simulink model "ROPOD_4Wheel_Tdistkinb_cntr"  (R2017b)
settings: Solver=ode1  StartTime=0.0  StopTime=Tfinal  FixedStep=Ts  RelTol=1e-3  EnableMultiTasking=on
PreLoadFcn:
  | init_model
InitFcn:
  | init_model
values from neighbouring files (symbols this model uses):
  FFtheta_intia = 0    [init_model.m]
  FFxy_mass = 0*80    (= 0)    [init_model.m]
  I_fhz_dtheta_cntr = 0.3    [init_model.m]
  I_fhz_dxdy_cntr = 0.25    [init_model.m]
  K_gain_dtheta_cntr = 150    [init_model.m]
  K_gain_dxdy_cntr = 200    [init_model.m]
  LL_wp_fhz_dtheta_cntr = 20    [init_model.m]
  LL_wp_fhz_dxdy_cntr = 20    [init_model.m]
  LL_wz_fhz_dtheta_cntr = 20    [init_model.m]
  LL_wz_fhz_dxdy_cntr = 20    [init_model.m]
  LPF_fhz_ddelta_meas = 50    [init_model.m]
  LPF_fhz_dtheta_cntr = 100    [init_model.m]
  LPF_fhz_dvarphi_meas = 50    [init_model.m]
  LPF_fhz_dxdy_cntr = 100    [init_model.m]
  max_hw_tau = 7.0    (= 7)    [init_model.m]
  max_ropod_acc_theta = 1.6    [init_model.m]
  max_ropod_acc_xy = 2.0    (= 2)    [init_model.m]
  max_ropod_sw_force = 500    [init_model.m]
  max_ropod_sw_tau = 250    [init_model.m]
  max_ropod_vel_theta = 1.6    [init_model.m]
  max_ropod_vel_xy = 2.0    (= 2)    [init_model.m]
  max_sw_current = 10    [init_model.m]
  Nwheels = 4    [Jqwl_numeric_function.m]    (also in S_matrix.m; extract_kinmodel_parameters.m; init_model.m; tau_optimal_dist_vec_fun.m)
  pivot_offs_sws = [3.835 3.465 2.059 0.357]    [init_model.m]
  ropod_kinmodel_pv = struct2array(ropod_kinmodel_param)    [set_ropod_KinModparams.m]
  SW_COM1_ENABLE1 = hex2dec('0001')    [init_model.m]
  SW_COM1_ENABLE2 = hex2dec('0002')    [init_model.m]
  SW_COM1_MODE_TORQUE = bitshift(hex2dec('0000'),2)    [init_model.m]
  SW_COM1_MODE_VELOCITY = bitshift(hex2dec('0002'),2)    [init_model.m]
  SW_COM1_USE_TS = hex2dec('8000')    [init_model.m]
  sw_tau_2_curr = 1/motor_physical_parameters.torqueconstant.value    [init_model.m]
  Taucompfactor = 2.0    (= 2)    [init_model.m]
  Tinit = 0*Tslot    [init_model.m]
  Ts = 0.001    [init_model.m]
undefined symbols (not defined in the file or in its folder): DiscIntNeverNeededParam, I_fhz_dvarphi_cntr, K_gain_dvarphi_cntr, LL_wp_fhz_dvarphi_cntr, LL_wz_fhz_dvarphi_cntr, LPF_fhz_dvarphi_cntr
libraries: simulink x37, cstblocks x23, dspsigops x12, SOEM_EtherCAT_Lib x5
(part 1 of 3)
settings Model: SimulationMode=external  Creator=cesar  LastModifiedBy=cesar
settings OptimizationCC: PassReuseOutputArgsThreshold=0  MaxStackSize=64
settings DebuggingCC: ParameterTunabilityLossMsg=error
settings HardwareCC: ProdBitPerLong=64  ProdHWDeviceType=Intel->x86-64 (Linux 64)  TargetBitPerLong=64  TargetBitPerPointer=64  TargetBitPerSizeT=64  TargetBitPerPtrDiffT=64  TargetLargestAtomicFloat=Float  TargetIntDivRoundTo=Zero  TargetEndianess=LittleEndian  TargetWordSize=64  TargetHWDeviceType=Intel->x86-64 (Linux 64)
settings SFSimCC: MATLABDynamicMemAlloc=off
settings RTWCC: SystemTargetFile=mttarget.tlc  MakeCommand="make_rtw  CC=\"ccache gcc\" OPTS=\"-DNETIF_ID=0 -DTEST_CONN_MODEL -D_GNU_SOURCE -DPRIO=99\""  TemplateMakefile=mt_unix.tmf  Description=Generic Real-Time Target  CustomInclude=/usr/local/include/soem  CustomLibrary=/usr/local/lib/libsoem.so  Toolchain=Catkin  BuildConfiguration=Faster Runs  RTWCompilerOptimization=Custom  RTWCustomCompilerOptimizations=-O2 -g -W
settings CodeAppCC: ForceParamTrailComments=on  OperatorAnnotations=on
settings GRTTargetCC: TargetLangStandard=C89/C90 (ANSI)  UseToolchainInfoCompliant=off  ExtMode=on

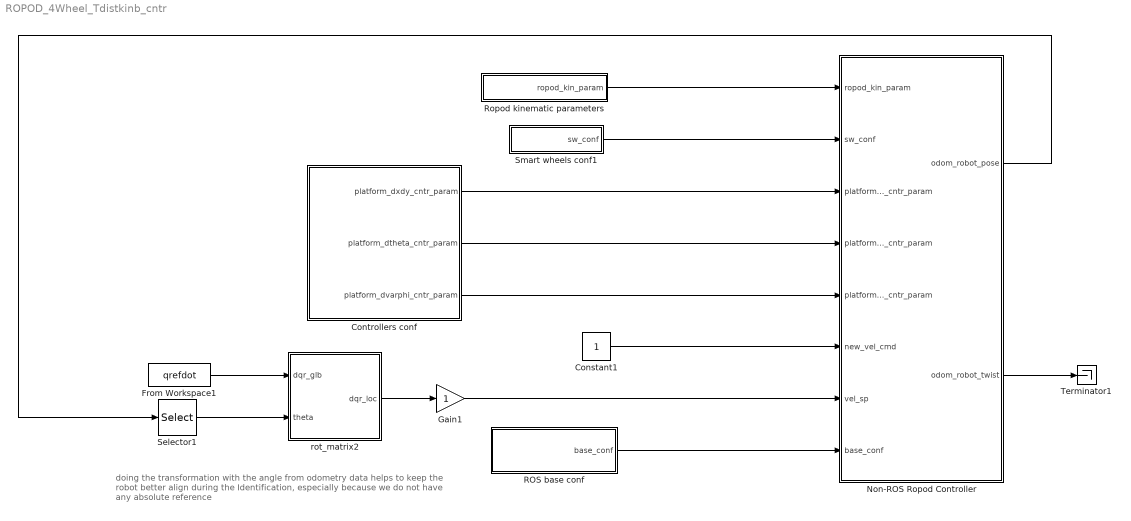
== system ROPOD_4Wheel_Tdistkinb_cntr ==
  note: doing the transformation with the angle from odometry data helps
      | to keep the robot better align during the Identification, especially because
      | we do not have any absolute reference
  Constant1 : Constant
  Controllers conf : Subsystem
  From Workspace1 : FromWorkspace  VariableName=qrefdot  SampleTime=0
  Gain1 : Gain
  Non-ROS Ropod Controller : Subsystem
  ROS base conf : Subsystem
  Ropod kinematic parameters : Subsystem
  Selector1 : Selector  InputPortWidth=3  IndexOptions=Index vector (dialog)  Indices=3  OutputSizes=1
  Smart wheels conf1 : Subsystem
  Terminator1 : Terminator
  rot_matrix2 : MATLAB Function  TreatAsAtomicUnit=on
  wires:
  Non-ROS Ropod Controller/1(odom_robot_pose) -> Selector1/1
  Gain1/1 -> Non-ROS Ropod Controller/7(vel_sp)
  ROS base conf/1(base_conf) -> Non-ROS Ropod Controller/8(base_conf)
  Non-ROS Ropod Controller/2(odom_robot_twist) -> Terminator1/1
  Constant1/1 -> Non-ROS Ropod Controller/6(new_vel_cmd)
  Controllers conf/1(platform_dxdy_cntr_param) -> Non-ROS Ropod Controller/3(platform_dxdy_cntr_param)
  Smart wheels conf1/1(sw_conf) -> Non-ROS Ropod Controller/2(sw_conf)
  Ropod kinematic parameters/1(ropod_kin_param) -> Non-ROS Ropod Controller/1(ropod_kin_param)
  From Workspace1/1 -> rot_matrix2/1(dqr_glb)
  Controllers conf/3(platform_dvarphi_cntr_param) -> Non-ROS Ropod Controller/5(platform_dvarphi_cntr_param)
  rot_matrix2/1(dqr_loc) -> Gain1/1
  Selector1/1 -> rot_matrix2/2(theta)
  Controllers conf/2(platform_dtheta_cntr_param) -> Non-ROS Ropod Controller/4(platform_dtheta_cntr_param)

== system ROPOD_4Wheel_Tdistkinb_cntr/Controllers conf ==
  Bus Creator : BusCreator  Inputs=5
  Bus Creator1 : BusCreator  Inputs=5
  Bus Creator2 : BusCreator  Inputs=5
  Constant1 : Constant  Value=I_fhz_dxdy_cntr
  Constant10 : Constant  Value=K_gain_dtheta_cntr
  Constant11 : Constant  Value=K_gain_dvarphi_cntr
  Constant12 : Constant  Value=I_fhz_dvarphi_cntr
  Constant13 : Constant  Value=LL_wp_fhz_dvarphi_cntr
  Constant14 : Constant  Value=LL_wz_fhz_dvarphi_cntr
  Constant15 : Constant  Value=LPF_fhz_dvarphi_cntr
  Constant2 : Constant  Value=LL_wp_fhz_dxdy_cntr
  Constant3 : Constant  Value=LL_wz_fhz_dxdy_cntr
  Constant4 : Constant  Value=LPF_fhz_dxdy_cntr
  Constant5 : Constant  Value=I_fhz_dtheta_cntr
  Constant6 : Constant  Value=LL_wp_fhz_dtheta_cntr
  Constant7 : Constant  Value=K_gain_dxdy_cntr
  Constant8 : Constant  Value=LL_wz_fhz_dtheta_cntr
  Constant9 : Constant  Value=LPF_fhz_dtheta_cntr
  platform_dxdy_cntr_param : Outport
  platform_dtheta_cntr_param : Outport  Port=2
  platform_dvarphi_cntr_param : Outport  Port=3
  wires:
  Constant2/1 -> Bus Creator/4  "LL_pole_fhz"
  Constant4/1 -> Bus Creator/5  "LPF_fhz"
  Bus Creator/1 -> platform_dxdy_cntr_param/1
  Constant1/1 -> Bus Creator/2  "I_freq_hz"
  Constant3/1 -> Bus Creator/3  "LL_zero_fhz"
  Constant7/1 -> Bus Creator/1  "P_gain"
  Bus Creator1/1 -> platform_dtheta_cntr_param/1
  Bus Creator2/1 -> platform_dvarphi_cntr_param/1
  Constant5/1 -> Bus Creator1/2  "I_freq_hz"
  Constant6/1 -> Bus Creator1/4  "LL_pole_fhz"
  Constant10/1 -> Bus Creator1/1  "P_gain"
  Constant8/1 -> Bus Creator1/3  "LL_zero_fhz"
  Constant9/1 -> Bus Creator1/5  "LPF_fhz"
  Constant15/1 -> Bus Creator2/5  "LPF_fhz"
  Constant12/1 -> Bus Creator2/2  "I_freq_hz"
  Constant14/1 -> Bus Creator2/3  "LL_zero_fhz"
  Constant11/1 -> Bus Creator2/1  "P_gain"
  Constant13/1 -> Bus Creator2/4  "LL_pole_fhz"

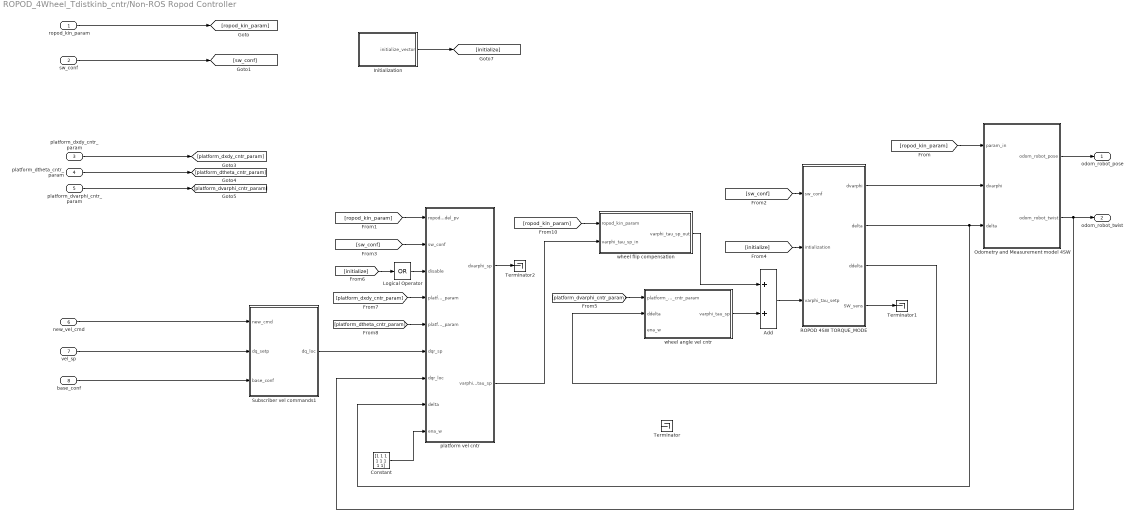
== system ROPOD_4Wheel_Tdistkinb_cntr/Non-ROS Ropod Controller ==
  ropod_kin_param : Inport
  sw_conf : Inport  Port=2
  platform_dxdy_cntr_param : Inport  Port=3
  platform_dtheta_cntr_param : Inport  Port=4
  platform_dvarphi_cntr_param : Inport  Port=5
  new_vel_cmd : Inport  Port=6
  vel_sp : Inport  Port=7
  base_conf : Inport  Port=8
  Add : Sum
  Constant : Constant  Value=[1 1 1 1 1 1 1 1]
  Initialization : Subsystem
  Logical Operator : Logic  Operator=OR  Inputs=1  AllPortsSameDT=off  OutDataTypeStr=boolean
  Odometry and Measurement model 4SW : Subsystem
  ROPOD 4SW TORQUE_MODE : Subsystem
  Subscriber vel commands1 : Subsystem
  Terminator : Terminator
  Terminator1 : Terminator
  Terminator2 : Terminator
  platform vel cntr : Subsystem
  wheel angle vel cntr : Subsystem
  wheel flip compensation : Subsystem
  odom_robot_pose : Outport
  odom_robot_twist : Outport  Port=2
  wires:
  sw_conf/1 -> [sw_conf]
  platform_dvarphi_cntr_param/1 -> [platform_dvarphi_cntr_param]
  platform_dxdy_cntr_param/1 -> [platform_dxdy_cntr_param]
  ropod_kin_param/1 -> [ropod_kin_param]
  platform_dtheta_cntr_param/1 -> [platform_dtheta_cntr_param]
  [ropod_kin_param] -> platform vel cntr/1(ropod_kinmodel_pv)
  Add/1 -> ROPOD 4SW TORQUE_MODE/3(varphi_tau_setp)
  ROPOD 4SW TORQUE_MODE/2(delta) -> platform vel cntr/8(delta), Odometry and Measurement model 4SW/3(delta)
  vel_sp/1 -> Subscriber vel commands1/2(dq_setp)
  ROPOD 4SW TORQUE_MODE/3(ddelta) -> wheel angle vel cntr/2(ddelta)
  [initialize] -> Logical Operator/1
  platform vel cntr/2(varphi_tau_sp) -> wheel flip compensation/2(varphi_tau_sp_in)
  Odometry and Measurement model 4SW/2(odom_robot_twist) -> odom_robot_twist/1, platform vel cntr/7(dqr_loc)
  [sw_conf] -> ROPOD 4SW TORQUE_MODE/1(sw_conf)
  Subscriber vel commands1/1(dq_loc) -> platform vel cntr/6(dqr_sp)
  ROPOD 4SW TORQUE_MODE/4(SW_sens) -> Terminator1/1
  base_conf/1 -> Subscriber vel commands1/3(base_conf)
  ROPOD 4SW TORQUE_MODE/1(dvarphi) -> Odometry and Measurement model 4SW/2(dvarphi)
  [ropod_kin_param] -> Odometry and Measurement model 4SW/1(param_in)
  Constant/1 -> platform vel cntr/9(ena_w)
  Odometry and Measurement model 4SW/1(odom_robot_pose) -> odom_robot_pose/1
  new_vel_cmd/1 -> Subscriber vel commands1/1(new_cmd)
  [platform_dtheta_cntr_param] -> platform vel cntr/5(platform_dtheta_cntr_param)
  [platform_dxdy_cntr_param] -> platform vel cntr/4(platform_dxdy_cntr_param)
  [sw_conf] -> platform vel cntr/2(sw_conf)
  [initialize] -> ROPOD 4SW TORQUE_MODE/2(intialization)
  Initialization/1(initialize_vector) -> [initialize]
  Logical Operator/1 -> platform vel cntr/3(disable)
  platform vel cntr/1(dvarphi_sp) -> Terminator2/1
  wheel angle vel cntr/1(varphi_tau_sp) -> Add/2
  [ropod_kin_param] -> wheel flip compensation/1(ropod_kin_param)
  wheel flip compensation/1(varphi_tau_sp_out) -> Add/1
  [platform_dvarphi_cntr_param] -> wheel angle vel cntr/1(platform_ddelta_cntr_param)

== system ROPOD_4Wheel_Tdistkinb_cntr/ROS base conf ==
  Bus Creator : BusCreator  Inputs=4
  max_ropod_acc_theta : Constant  Value=max_ropod_acc_theta
  max_ropod_acc_xy : Constant  Value=max_ropod_acc_xy
  max_ropod_vel_theta : Constant  Value=max_ropod_vel_theta
  max_ropod_vel_xy : Constant  Value=max_ropod_vel_xy
  base_conf : Outport
  wires:
  max_ropod_acc_xy/1 -> Bus Creator/2  "max_acc_xy"
  max_ropod_vel_xy/1 -> Bus Creator/1  "max_vel_xy"
  Bus Creator/1 -> base_conf/1
  max_ropod_acc_theta/1 -> Bus Creator/4  "max_acc_theta"
  max_ropod_vel_theta/1 -> Bus Creator/3  "max_vel_theta"

== system ROPOD_4Wheel_Tdistkinb_cntr/Ropod kinematic parameters ==
  ropod_kinmodel_pv : Constant  Value=ropod_kinmodel_pv
  ropod_kin_param : Outport
  wires:
  ropod_kinmodel_pv/1 -> ropod_kin_param/1

== system ROPOD_4Wheel_Tdistkinb_cntr/Smart wheels conf1 ==
  Bus Creator : BusCreator  Inputs=8
  LPF_fhz_ddelta_meas : Constant  Value=LPF_fhz_ddelta_meas
  LPF_fhz_dvarphi_meas : Constant  Value=LPF_fhz_dvarphi_meas
  enable : Constant
  max_current : Constant  Value=max_sw_current
  pivot_offset_sw1 : Constant  Value=pivot_offs_sws(1)
  pivot_offset_sw2 : Constant  Value=pivot_offs_sws(2)
  pivot_offset_sw3 : Constant  Value=pivot_offs_sws(3)
  pivot_offset_sw4 : Constant  Value=pivot_offs_sws(4)
  sw_conf : Outport
  wires:
  enable/1 -> Bus Creator/1  "enable"
  Bus Creator/1 -> sw_conf/1
  max_current/1 -> Bus Creator/2  "max_current"
  pivot_offset_sw1/1 -> Bus Creator/3  "pivot_offs_sw1"
  pivot_offset_sw2/1 -> Bus Creator/4  "pivot_offs_sw2"
  pivot_offset_sw3/1 -> Bus Creator/5  "pivot_offs_sw3"
  pivot_offset_sw4/1 -> Bus Creator/6  "pivot_offs_sw4"
  LPF_fhz_dvarphi_meas/1 -> Bus Creator/7  "dvarphi_LPF_fhz"
  LPF_fhz_ddelta_meas/1 -> Bus Creator/8  "ddelta_LPF_fhz"

== system ROPOD_4Wheel_Tdistkinb_cntr/Non-ROS Ropod Controller/Initialization ==
  note: Allow Tinit/Nwheels seconds for initialization per wheel
  Digital Clock : DigitalClock  SampleTime=Ts
  Logical Operator : Logic  AllPortsSameDT=off  OutDataTypeStr=boolean
  Logical Operator1 : Logic  Operator=NOT  AllPortsSameDT=off  OutDataTypeStr=boolean
  Logical Operator2 : Logic  Operator=NOT  AllPortsSameDT=off  OutDataTypeStr=boolean
  Logical Operator3 : Logic  AllPortsSameDT=off  OutDataTypeStr=boolean
  Logical Operator4 : Logic  Operator=NOT  AllPortsSameDT=off  OutDataTypeStr=boolean
  Logical Operator5 : Logic  AllPortsSameDT=off  OutDataTypeStr=boolean
  Mux : Mux
  comp : simulink/Logic and Bit Operations/Compare To Constant  relop=<  const=Tinit/Nwheels  OutDataTypeStr=boolean
  comp1 : simulink/Logic and Bit Operations/Compare To Constant  relop=<  const=2*Tinit/Nwheels  OutDataTypeStr=boolean
  comp2 : simulink/Logic and Bit Operations/Compare To Constant  relop=<  const=3*Tinit/Nwheels  OutDataTypeStr=boolean
  comp3 : simulink/Logic and Bit Operations/Compare To Constant  relop=<  const=4*Tinit/Nwheels  OutDataTypeStr=boolean
  initialize_vector : Outport
  wires:
  Logical Operator5/1 -> Mux/4
  Logical Operator3/1 -> Mux/3
  comp3/1 -> Logical Operator5/2
  Logical Operator2/1 -> Logical Operator3/1
  Logical Operator1/1 -> Logical Operator/1
  Logical Operator4/1 -> Logical Operator5/1
  Mux/1 -> initialize_vector/1
  comp/1 -> Logical Operator1/1, Mux/1
  comp1/1 -> Logical Operator2/1, Logical Operator/2
  Logical Operator/1 -> Mux/2
  comp2/1 -> Logical Operator4/1, Logical Operator3/2
  Digital Clock/1 -> comp3/1, comp2/1, comp1/1, comp/1

== system ROPOD_4Wheel_Tdistkinb_cntr/Non-ROS Ropod Controller/Odometry and Measurement model 4SW ==
  note: This output is only useful when using ros
      | This data is fed to /odom/pose
  note: This part is in global coordinates
  note: This part is in local coordinates
  param_in : Inport
  dvarphi : Inport  Port=2
  delta : Inport  Port=3
  Discrete-Time Integrator : DiscreteIntegrator  InitialConditionSetting=State (most efficient)  SampleTime=Ts  ICPrevOutput=DiscIntNeverNeededParam  ICPrevScaledInput=DiscIntNeverNeededParam
  Jqwl_matrix : MATLAB Function  TreatAsAtomicUnit=on
  Product3 : Product  Multiplication=Matrix(*)
  Selector3 : Selector  InputPortWidth=3  IndexOptions=Index vector (dialog)  Indices=3  OutputSizes=1
  Signal Specification : SignalSpecification  Dimensions=[3 1]
  pos_rot_matrix : MATLAB Function  TreatAsAtomicUnit=on
  odom_robot_pose : Outport
  odom_robot_twist : Outport  Port=2
  wires:
  Product3/1 -> Signal Specification/1
  param_in/1 -> Jqwl_matrix/1(ropod_kinmodel_param_vec)
  delta/1 -> Jqwl_matrix/2(delta)
  Jqwl_matrix/1(Jqwl) -> Product3/1
  dvarphi/1 -> Product3/2
  Signal Specification/1 -> pos_rot_matrix/1(dqr_loc), odom_robot_twist/1
  Selector3/1 -> pos_rot_matrix/2(theta_odom)
  pos_rot_matrix/1(dqr_glb) -> Discrete-Time Integrator/1
  Discrete-Time Integrator/1 -> odom_robot_pose/1, Selector3/1

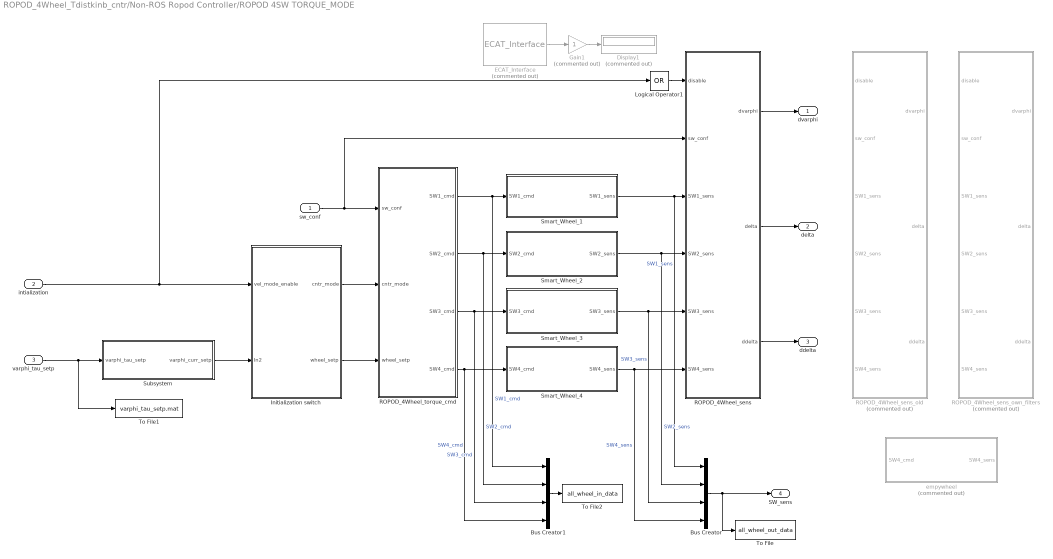
== system ROPOD_4Wheel_Tdistkinb_cntr/Non-ROS Ropod Controller/ROPOD 4SW TORQUE_MODE ==
  sw_conf : Inport
  intialization : Inport  Port=2
  varphi_tau_setp : Inport  Port=3
  Bus Creator : BusCreator  Inputs=4
  Bus Creator1 : BusCreator  Inputs=4
  Display1 : Display  Commented=on
  ECAT_Interface : SOEM_EtherCAT_Lib/ECAT_Interface  Priority=0  Commented=on  IFINTERFACE=eth0  TS=Ts
      settings: SourceProductName=SOEM_EtherCAT_Lib
  Gain1 : Gain  Commented=on  OutDataTypeStr=double
  Initialization switch : Subsystem
  Logical Operator1 : Logic  Operator=OR  Inputs=1  AllPortsSameDT=off  OutDataTypeStr=boolean
  ROPOD_4Wheel_sens : Subsystem
  ROPOD_4Wheel_sens_old : Subsystem  Commented=on
  ROPOD_4Wheel_sens_own_filters : Subsystem  Commented=on
  ROPOD_4Wheel_torque_cmd : Subsystem
  Smart_Wheel_1 : Subsystem
  Smart_Wheel_2 : Subsystem
  Smart_Wheel_3 : Subsystem
  Smart_Wheel_4 : Subsystem
  Subsystem : Subsystem
  To File : ToFile  Filename=all_wheel_out_data  MatrixName=all_wheel_out_data
  To File1 : ToFile  Filename=varphi_tau_setp.mat  MatrixName=varphi_tau_setp
  To File2 : ToFile  Filename=all_wheel_in_data  MatrixName=all_wheel_in_data
  empywheel : Subsystem  Commented=on
  dvarphi : Outport
  delta : Outport  Port=2
  ddelta : Outport  Port=3
  SW_sens : Outport  Port=4
  wires:
  ROPOD_4Wheel_sens/2(delta) -> delta/1
  ROPOD_4Wheel_sens/1(dvarphi) -> dvarphi/1
  ECAT_Interface/1 -> Gain1/1
  Gain1/1 -> Display1/1
  ROPOD_4Wheel_sens/3(ddelta) -> ddelta/1
  ROPOD_4Wheel_torque_cmd/4(SW4_cmd) -> Bus Creator1/4, Smart_Wheel_4/1(SW4_cmd)  "SW4_cmd"
  ROPOD_4Wheel_torque_cmd/1(SW1_cmd) -> Bus Creator1/1, Smart_Wheel_1/1(SW1_cmd)  "SW1_cmd"
  ROPOD_4Wheel_torque_cmd/3(SW3_cmd) -> Bus Creator1/3, Smart_Wheel_3/1(SW3_cmd)  "SW3_cmd"
  sw_conf/1 -> ROPOD_4Wheel_sens/2(sw_conf), ROPOD_4Wheel_torque_cmd/1(sw_conf)
  ROPOD_4Wheel_torque_cmd/2(SW2_cmd) -> Bus Creator1/2, Smart_Wheel_2/1(SW2_cmd)  "SW2_cmd"
  Smart_Wheel_1/1(SW1_sens) -> ROPOD_4Wheel_sens/3(SW1_sens), Bus Creator/1  "SW1_sens"
  Smart_Wheel_4/1(SW4_sens) -> ROPOD_4Wheel_sens/6(SW4_sens), Bus Creator/4  "SW4_sens"
  Smart_Wheel_2/1(SW2_sens) -> ROPOD_4Wheel_sens/4(SW2_sens), Bus Creator/2  "SW2_sens"
  Smart_Wheel_3/1(SW3_sens) -> ROPOD_4Wheel_sens/5(SW3_sens), Bus Creator/3  "SW3_sens"
  Bus Creator/1 -> To File/1, SW_sens/1
  Initialization switch/1(cntr_mode) -> ROPOD_4Wheel_torque_cmd/2(cntr_mode)
  Initialization switch/2(wheel_setp) -> ROPOD_4Wheel_torque_cmd/3(wheel_setp)
  Subsystem/1(varphi_curr_setp) -> Initialization switch/2(In2)
  varphi_tau_setp/1 -> To File1/1, Subsystem/1(varphi_tau_setp)
  intialization/1 -> Logical Operator1/1, Initialization switch/1(vel_mode_enable)
  Bus Creator1/1 -> To File2/1
  Logical Operator1/1 -> ROPOD_4Wheel_sens/1(disable)

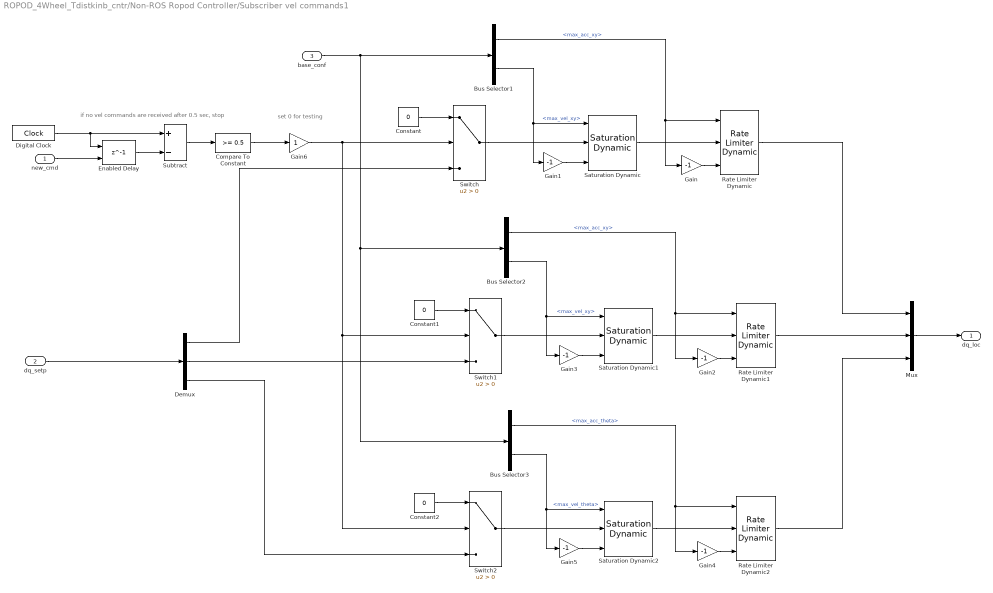
== system ROPOD_4Wheel_Tdistkinb_cntr/Non-ROS Ropod Controller/Subscriber vel commands1 ==
  note: set 0 for testing
  note: if no vel commands are received after 0.5 sec, stop
  new_cmd : Inport
  dq_setp : Inport  Port=2
  base_conf : Inport  Port=3
  Bus Selector1 : BusSelector  OutputSignals=max_acc_xy,max_vel_xy
  Bus Selector2 : BusSelector  OutputSignals=max_acc_xy,max_vel_xy
  Bus Selector3 : BusSelector  OutputSignals=max_acc_theta,max_vel_theta
  Compare To Constant : simulink/Logic and Bit Operations/Compare To Constant  relop=>=  const=0.5  OutDataTypeStr=boolean
  Constant : Constant  Value=0  SampleTime=Ts
  Constant1 : Constant  Value=0
  Constant2 : Constant  Value=0
  Demux : Demux  Outputs=3
  Digital Clock : DigitalClock  SampleTime=Ts
  Enabled Delay : Delay  DelayLength=1  ShowEnablePort=on  SampleTime=Ts
      settings: InputPortMap=u0,e6
  Gain{,1..5} (6 alike) : Gain  Gain=-1
  Gain6 : Gain
  Mux : Mux  Inputs=3
  Rate Limiter Dynamic : simulink/Discontinuities/Rate Limiter Dynamic
      settings: SourceProductName=Simulink
  Rate Limiter Dynamic1 : simulink/Discontinuities/Rate Limiter Dynamic
      settings: SourceProductName=Simulink
  Rate Limiter Dynamic2 : simulink/Discontinuities/Rate Limiter Dynamic
      settings: SourceProductName=Simulink
  Saturation Dynamic : simulink/Discontinuities/Saturation Dynamic  OutMin=[]  OutMax=[]  OutDataTypeStr=Inherit: Same as second input  OutDataType=fixdt(1, 16)  OutScaling=2^-10  DoSatur=off
  Saturation Dynamic1 : simulink/Discontinuities/Saturation Dynamic  OutMin=[]  OutMax=[]  OutDataTypeStr=Inherit: Same as second input  OutDataType=fixdt(1, 16)  OutScaling=2^-10  DoSatur=off
  Saturation Dynamic2 : simulink/Discontinuities/Saturation Dynamic  OutMin=[]  OutMax=[]  OutDataTypeStr=Inherit: Same as second input  OutDataType=fixdt(1, 16)  OutScaling=2^-10  DoSatur=off
  Subtract : Sum  Inputs=+-
  Switch : Switch  Criteria=u2 > Threshold
  Switch1 : Switch  Criteria=u2 > Threshold
  Switch2 : Switch  Criteria=u2 > Threshold
  dq_loc : Outport
  wires:
  Demux/1 -> Switch/3
  dq_setp/1 -> Demux/1
  new_cmd/1 -> Enabled Delay/2
  Digital Clock/1 -> Enabled Delay/1, Subtract/1
  Enabled Delay/1 -> Subtract/2
  Subtract/1 -> Compare To Constant/1
  Constant/1 -> Switch/1
  Gain/1 -> Rate Limiter Dynamic/3
  Switch/1 -> Saturation Dynamic/2
  Gain1/1 -> Saturation Dynamic/3
  Saturation Dynamic/1 -> Rate Limiter Dynamic/2
  Switch1/1 -> Saturation Dynamic1/2
  Gain3/1 -> Saturation Dynamic1/3
  Constant1/1 -> Switch1/1
  Demux/2 -> Switch1/3
  Gain2/1 -> Rate Limiter Dynamic1/3
  Saturation Dynamic1/1 -> Rate Limiter Dynamic1/2
  Bus Selector2/1 -> Rate Limiter Dynamic1/1, Gain2/1  "<max_acc_xy>"
  Bus Selector2/2 -> Saturation Dynamic1/1, Gain3/1  "<max_vel_xy>"
  Bus Selector3/1 -> Rate Limiter Dynamic2/1, Gain4/1  "<max_acc_theta>"
  Saturation Dynamic2/1 -> Rate Limiter Dynamic2/2
  base_conf/1 -> Bus Selector3/1, Bus Selector2/1, Bus Selector1/1
  Switch2/1 -> Saturation Dynamic2/2
  Constant2/1 -> Switch2/1
  Demux/3 -> Switch2/3
  Gain5/1 -> Saturation Dynamic2/3
  Gain4/1 -> Rate Limiter Dynamic2/3
  Compare To Constant/1 -> Gain6/1
  Bus Selector3/2 -> Saturation Dynamic2/1, Gain5/1  "<max_vel_theta>"
  Mux/1 -> dq_loc/1
  Rate Limiter Dynamic/1 -> Mux/1
  Rate Limiter Dynamic1/1 -> Mux/2
  Rate Limiter Dynamic2/1 -> Mux/3
  Bus Selector1/2 -> Saturation Dynamic/1, Gain1/1  "<max_vel_xy>"
  Bus Selector1/1 -> Rate Limiter Dynamic/1, Gain/1  "<max_acc_xy>"
  Gain6/1 -> Switch2/2, Switch1/2, Switch/2

== system ROPOD_4Wheel_Tdistkinb_cntr/Non-ROS Ropod Controller/platform vel cntr ==
  ropod_kinmodel_pv : Inport
  sw_conf : Inport  Port=2
  disable : Inport  Port=3
  platform_dxdy_cntr_param : Inport  Port=4
  platform_dtheta_cntr_param : Inport  Port=5
  dqr_sp : Inport  Port=6
  dqr_loc : Inport  Port=7
  delta : Inport  Port=8
  ena_w : Inport  Port=9
  Inverse Kinematics 4SW : Subsystem
  Platorm Velocity controller : Subsystem
  Torque distribution : Subsystem
  dvarphi_sp : Outport
  varphi_tau_sp : Outport  Port=2
  wires:
  delta/1 -> Torque distribution/5(delta), Inverse Kinematics 4SW/3(delta)
  ena_w/1 -> Torque distribution/4(ena_w)
  sw_conf/1 -> Torque distribution/3(sw_conf)
  Torque distribution/1(varphi_tau_setp_out) -> varphi_tau_sp/1
  ropod_kinmodel_pv/1 -> Inverse Kinematics 4SW/1(param_in), Torque distribution/2(ropod_kinmodel_pv)
  Platorm Velocity controller/1(f_body_setp) -> Torque distribution/1(tau_body)
  disable/1 -> Platorm Velocity controller/1(reset_int)
  dqr_sp/1 -> Platorm Velocity controller/2(dqr_sp), Inverse Kinematics 4SW/2(dqr_sp)
  dqr_loc/1 -> Platorm Velocity controller/3(dqr_loc)
  Inverse Kinematics 4SW/1(wheel_vel_sp) -> dvarphi_sp/1
  platform_dxdy_cntr_param/1 -> Platorm Velocity controller/4(platform_dxdy_cntr_param)
  platform_dtheta_cntr_param/1 -> Platorm Velocity controller/5(platform_dtheta_cntr_param)

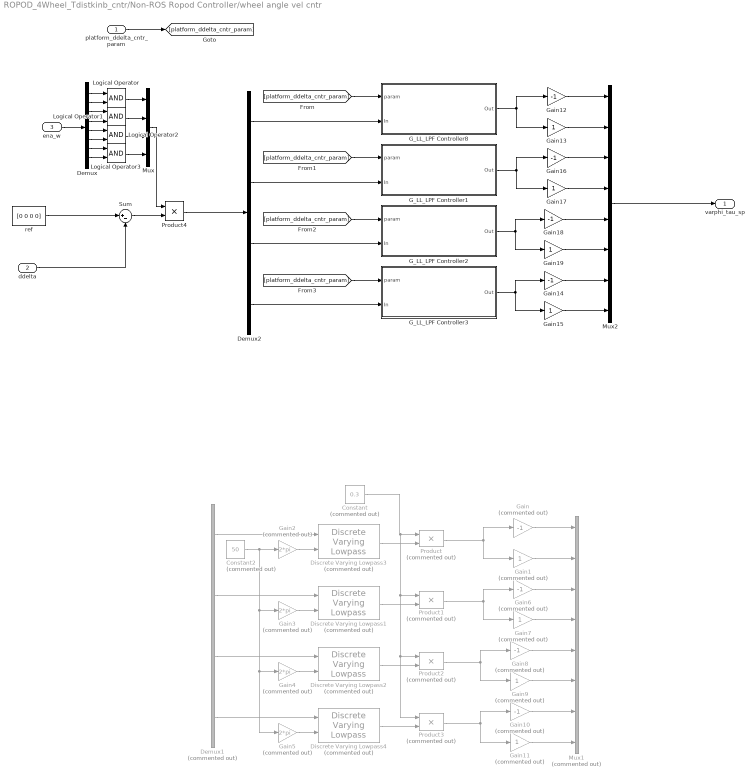
== system ROPOD_4Wheel_Tdistkinb_cntr/Non-ROS Ropod Controller/wheel angle vel cntr ==
  platform_ddelta_cntr_param : Inport
  ddelta : Inport  Port=2
  ena_w : Inport  Port=3
  Constant : Constant  Commented=on  Value=0.3
  Constant2 : Constant  Commented=on  Value=50
  Demux : Demux  Outputs=8
  Demux1 : Demux  Commented=on
  Demux2 : Demux
  Discrete Varying Lowpass{1..4} (4 alike) : cstblocks/Linear Parameter Varying/Discrete Varying Lowpass  Commented=on  N=1  w0=0  Ts=Ts
      settings: SourceProductName=Control System Toolbox  SourceProductBaseCode=CT
  G_LL_LPF Controller1 : Subsystem
  G_LL_LPF Controller2 : Subsystem
  G_LL_LPF Controller3 : Subsystem
  G_LL_LPF Controller8 : Subsystem
  Gain{,6,8,10} (4 alike) : Gain  Commented=on  Gain=-1
  Gain{1,7,9,11} (4 alike) : Gain  Commented=on
  Gain{12,14,16,18} (4 alike) : Gain  Gain=-1
  Gain{13,15,17,19} (4 alike) : Gain
  Gain{2..5} (4 alike) : Gain  Commented=on  Gain=2*pi
  Logical Operator{,1..3} (4 alike) : Logic  AllPortsSameDT=off  OutDataTypeStr=boolean
  Mux : Mux
  Mux1 : Mux  Commented=on  Inputs=8
  Mux2 : Mux  Inputs=8
  Product{,1..3} (4 alike) : Product  Commented=on
  Product4 : Product
  Sum : Sum  Inputs=|+-
  ref : Constant  Value=[0 0 0 0]
  varphi_tau_sp : Outport
  wires:
  ddelta/1 -> Sum/2
  ref/1 -> Sum/1
  Mux2/1 -> varphi_tau_sp/1
  Product1/1 -> Gain6/1, Gain7/1
  Gain3/1 -> Discrete Varying Lowpass1/2
  Constant2/1 -> Gain5/1, Gain4/1, Gain3/1, Gain2/1
  Product/1 -> Gain1/1, Gain/1
  Product2/1 -> Gain9/1, Gain8/1
  Gain6/1 -> Mux1/3
  Discrete Varying Lowpass4/1 -> Product3/2
  Demux1/1 -> Discrete Varying Lowpass3/1
  Discrete Varying Lowpass2/1 -> Product2/2
  Demux1/3 -> Discrete Varying Lowpass2/1
  Discrete Varying Lowpass3/1 -> Product/2
  Gain5/1 -> Discrete Varying Lowpass4/2
  Gain4/1 -> Discrete Varying Lowpass2/2
  Constant/1 -> Product3/1, Product2/1, Product1/1, Product/1
  Gain8/1 -> Mux1/5
  Gain9/1 -> Mux1/6
  Gain/1 -> Mux1/1
  Product3/1 -> Gain11/1, Gain10/1
  Gain7/1 -> Mux1/4
  Discrete Varying Lowpass1/1 -> Product1/2
  Demux1/2 -> Discrete Varying Lowpass1/1
  Gain11/1 -> Mux1/8
  Gain1/1 -> Mux1/2
  Demux1/4 -> Discrete Varying Lowpass4/1
  Gain10/1 -> Mux1/7
  Gain2/1 -> Discrete Varying Lowpass3/2
  G_LL_LPF Controller8/1(Out) -> Gain13/1, Gain12/1
  Gain14/1 -> Mux2/7
  Gain18/1 -> Mux2/5
  G_LL_LPF Controller1/1(Out) -> Gain16/1, Gain17/1
  Gain15/1 -> Mux2/8
  Gain16/1 -> Mux2/3
  G_LL_LPF Controller2/1(Out) -> Gain19/1, Gain18/1
  Gain19/1 -> Mux2/6
  G_LL_LPF Controller3/1(Out) -> Gain15/1, Gain14/1
  Gain13/1 -> Mux2/2
  Gain12/1 -> Mux2/1
  Gain17/1 -> Mux2/4
  platform_ddelta_cntr_param/1 -> [platform_ddelta_cntr_param]
  [platform_ddelta_cntr_param] -> G_LL_LPF Controller8/1(param)
  Demux2/1 -> G_LL_LPF Controller8/2(In)
  Demux2/2 -> G_LL_LPF Controller1/2(In)
  Demux2/3 -> G_LL_LPF Controller2/2(In)
  Demux2/4 -> G_LL_LPF Controller3/2(In)
  [platform_ddelta_cntr_param] -> G_LL_LPF Controller1/1(param)
  [platform_ddelta_cntr_param] -> G_LL_LPF Controller2/1(param)
  [platform_ddelta_cntr_param] -> G_LL_LPF Controller3/1(param)
  ena_w/1 -> Demux/1
  Demux/1 -> Logical Operator/1
  Demux/2 -> Logical Operator/2
  Logical Operator/1 -> Mux/1
  Demux/3 -> Logical Operator1/1
  Demux/4 -> Logical Operator1/2
  Demux/5 -> Logical Operator2/1
  Demux/6 -> Logical Operator2/2
  Demux/7 -> Logical Operator3/1
  Demux/8 -> Logical Operator3/2
  Logical Operator1/1 -> Mux/2
  Logical Operator2/1 -> Mux/3
  Logical Operator3/1 -> Mux/4
  Mux/1 -> Product4/1
  Sum/1 -> Product4/2
  Product4/1 -> Demux2/1

== system ROPOD_4Wheel_Tdistkinb_cntr/Non-ROS Ropod Controller/wheel flip compensation ==
  ropod_kin_param : Inport
  varphi_tau_sp_in : Inport  Port=2
  Constant : Constant  Value=3
  Demux : Demux  Outputs=8
  MATLAB Function : MATLAB Function  TreatAsAtomicUnit=on
  MATLAB Function1 : MATLAB Function  TreatAsAtomicUnit=on
  MATLAB Function2 : MATLAB Function  TreatAsAtomicUnit=on
  MATLAB Function3 : MATLAB Function  TreatAsAtomicUnit=on
  Mux : Mux  Inputs=8
  Terminator : Terminator
  varphi_tau_sp_out : Outport
  wires:
  varphi_tau_sp_in/1 -> Demux/1
  ropod_kin_param/1 -> [ropod_kin_param]
  Constant/1 -> [kmax]
  Demux/2 -> MATLAB Function/2(tr)
  Demux/1 -> MATLAB Function/1(tl)
  [kmax] -> MATLAB Function/4(kmax)
  [ropod_kin_param] -> MATLAB Function/3(ropod_kinmodel_param_vec)
  Demux/4 -> MATLAB Function1/2(tr)
  Demux/3 -> MATLAB Function1/1(tl)
  [kmax] -> MATLAB Function1/4(kmax)
  [ropod_kin_param] -> MATLAB Function1/3(ropod_kinmodel_param_vec)
  Demux/6 -> MATLAB Function2/2(tr)
  Demux/5 -> MATLAB Function2/1(tl)
  [kmax] -> MATLAB Function2/4(kmax)
  [ropod_kin_param] -> MATLAB Function2/3(ropod_kinmodel_param_vec)
  Demux/8 -> MATLAB Function3/2(tr)
  Demux/7 -> MATLAB Function3/1(tl)
  [kmax] -> MATLAB Function3/4(kmax)
  [ropod_kin_param] -> MATLAB Function3/3(ropod_kinmodel_param_vec)
  MATLAB Function/1(tl_out) -> Mux/1
  MATLAB Function1/1(tl_out) -> Mux/3
  MATLAB Function2/1(tl_out) -> Mux/5
  MATLAB Function3/1(tl_out) -> Mux/7
  MATLAB Function/2(tr_out) -> Mux/2
  MATLAB Function1/2(tr_out) -> Mux/4
  MATLAB Function2/2(tr_out) -> Mux/6
  MATLAB Function3/2(tr_out) -> Mux/8
  MATLAB Function/3(sc) -> Terminator/1
  Mux/1 -> varphi_tau_sp_out/1

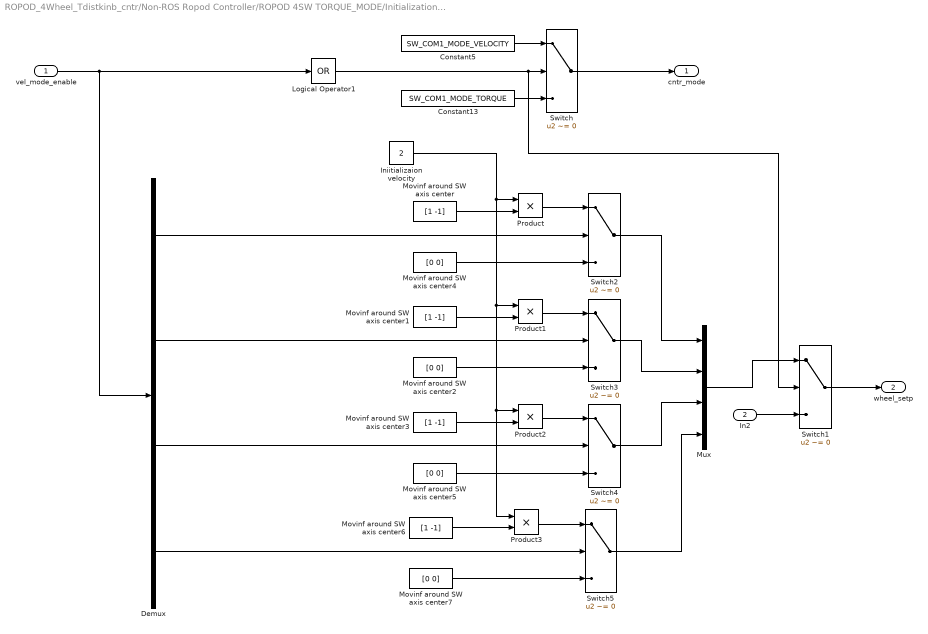
== system ROPOD_4Wheel_Tdistkinb_cntr/Non-ROS Ropod Controller/ROPOD 4SW TORQUE_MODE/Initialization switch ==
  vel_mode_enable : Inport
  In2 : Inport  Port=2
  Constant13 : Constant  Value=SW_COM1_MODE_TORQUE
  Constant5 : Constant  Value=SW_COM1_MODE_VELOCITY
  Demux : Demux
  Iniitializaion velocity : Constant  Value=2
  Logical Operator1 : Logic  Operator=OR  Inputs=1  AllPortsSameDT=off  OutDataTypeStr=boolean
  Movinf around SW axis center{,1,3,6} (4 alike) : Constant  Value=[1 -1]
  Movinf around SW axis center{2,4..5,7} (4 alike) : Constant  Value=[0 0]
  Mux : Mux
  Product{,1..3} (4 alike) : Product
  Switch{,1..5} (6 alike) : Switch  Criteria=u2 ~= 0
  cntr_mode : Outport
  wheel_setp : Outport  Port=2
  wires:
  Constant13/1 -> Switch/3
  Constant5/1 -> Switch/1
  vel_mode_enable/1 -> Demux/1, Logical Operator1/1
  Switch/1 -> cntr_mode/1
  Logical Operator1/1 -> Switch1/2, Switch/2
  Movinf around SW axis center/1 -> Product/2
  Iniitializaion velocity/1 -> Product3/1, Product2/1, Product1/1, Product/1
  Product/1 -> Switch2/1
  Movinf around SW axis center4/1 -> Switch2/3
  Demux/1 -> Switch2/2
  Movinf around SW axis center2/1 -> Switch3/3
  Movinf around SW axis center1/1 -> Product1/2
  Demux/2 -> Switch3/2
  Product1/1 -> Switch3/1
  Movinf around SW axis center5/1 -> Switch4/3
  Movinf around SW axis center3/1 -> Product2/2
  Demux/3 -> Switch4/2
  Product2/1 -> Switch4/1
  Movinf around SW axis center7/1 -> Switch5/3
  Movinf around SW axis center6/1 -> Product3/2
  Demux/4 -> Switch5/2
  Product3/1 -> Switch5/1
  Switch2/1 -> Mux/1
  Switch3/1 -> Mux/2
  Switch4/1 -> Mux/3
  Switch5/1 -> Mux/4
  In2/1 -> Switch1/3
  Mux/1 -> Switch1/1
  Switch1/1 -> wheel_setp/1

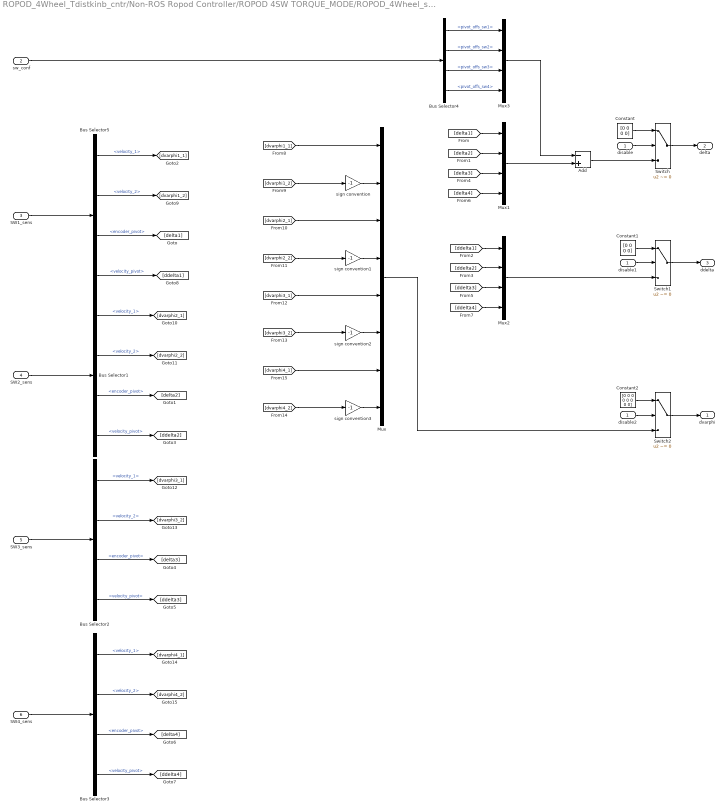
== system ROPOD_4Wheel_Tdistkinb_cntr/Non-ROS Ropod Controller/ROPOD 4SW TORQUE_MODE/ROPOD_4Wheel_sens ==
  disable : Inport
  sw_conf : Inport  Port=2
  SW1_sens : Inport  Port=3
  SW2_sens : Inport  Port=4
  SW3_sens : Inport  Port=5
  SW4_sens : Inport  Port=6
  Add : Sum  Inputs=-+
  Bus Selector{1..3,5} (4 alike) : BusSelector  OutputSignals=velocity_1,velocity_2,encoder_pivot,velocity_pivot
  Bus Selector4 : BusSelector  OutputSignals=pivot_offs_sw1,pivot_offs_sw2,pivot_offs_sw3,pivot_offs_sw4
  Constant : Constant  Value=[0 0 0 0]
  Constant1 : Constant  Value=[0 0 0 0]
  Constant2 : Constant  Value=[0 0 0 0 0 0 0 0]
  Mux : Mux  Inputs=8
  Mux1 : Mux
  Mux2 : Mux
  Mux3 : Mux
  Switch : Switch  Criteria=u2 ~= 0
  Switch1 : Switch  Criteria=u2 ~= 0
  Switch2 : Switch  Criteria=u2 ~= 0
  disable1 : InportShadow
  disable2 : InportShadow
  sign convention{,1..3} (4 alike) : Gain  Gain=-1
  dvarphi : Outport
  delta : Outport  Port=2
  ddelta : Outport  Port=3
  wires:
  SW1_sens/1 -> Bus Selector5/1
  [delta1] -> Mux1/1
  [delta2] -> Mux1/2
  [ddelta2] -> Mux2/2
  [ddelta1] -> Mux2/1
  [delta3] -> Mux1/3
  [ddelta3] -> Mux2/3
  [delta4] -> Mux1/4
  [ddelta4] -> Mux2/4
  Mux1/1 -> Add/2
  Mux3/1 -> Add/1
  Bus Selector4/1 -> Mux3/1  "<pivot_offs_sw1>"
  Bus Selector4/2 -> Mux3/2  "<pivot_offs_sw2>"
  Bus Selector4/3 -> Mux3/3  "<pivot_offs_sw3>"
  Bus Selector4/4 -> Mux3/4  "<pivot_offs_sw4>"
  sign convention/1 -> Mux/2
  sign convention1/1 -> Mux/4
  sign convention2/1 -> Mux/6
  sign convention3/1 -> Mux/8
  Add/1 -> Switch/3
  Switch/1 -> delta/1
  disable/1 -> Switch/2
  Constant/1 -> Switch/1
  Switch1/1 -> ddelta/1
  Mux2/1 -> Switch1/3
  Constant1/1 -> Switch1/1
  disable1/1 -> Switch1/2
  disable2/1 -> Switch2/2
  Constant2/1 -> Switch2/1
  Mux/1 -> Switch2/3
  Switch2/1 -> dvarphi/1
  Bus Selector5/4 -> [ddelta1]  "<velocity_pivot>"
  Bus Selector5/2 -> [dvarphi1_2]  "<velocity_2>"
  sw_conf/1 -> Bus Selector4/1
  [dvarphi1_1] -> Mux/1
  [dvarphi1_2] -> sign convention/1
  [dvarphi2_1] -> Mux/3
  [dvarphi2_2] -> sign convention1/1
  [dvarphi3_1] -> Mux/5
  [dvarphi3_2] -> sign convention2/1
  [dvarphi4_1] -> Mux/7
  [dvarphi4_2] -> sign convention3/1
  Bus Selector5/1 -> [dvarphi1_1]  "<velocity_1>"
  Bus Selector5/3 -> [delta1]  "<encoder_pivot>"
  SW2_sens/1 -> Bus Selector1/1
  Bus Selector1/4 -> [ddelta2]  "<velocity_pivot>"
  Bus Selector1/1 -> [dvarphi2_1]  "<velocity_1>"
  Bus Selector1/3 -> [delta2]  "<encoder_pivot>"
  Bus Selector1/2 -> [dvarphi2_2]  "<velocity_2>"
  Bus Selector2/2 -> [dvarphi3_2]  "<velocity_2>"
  Bus Selector2/1 -> [dvarphi3_1]  "<velocity_1>"
  Bus Selector2/4 -> [ddelta3]  "<velocity_pivot>"
  SW3_sens/1 -> Bus Selector2/1
  Bus Selector2/3 -> [delta3]  "<encoder_pivot>"
  Bus Selector3/3 -> [delta4]  "<encoder_pivot>"
  SW4_sens/1 -> Bus Selector3/1
  Bus Selector3/4 -> [ddelta4]  "<velocity_pivot>"
  Bus Selector3/1 -> [dvarphi4_1]  "<velocity_1>"
  Bus Selector3/2 -> [dvarphi4_2]  "<velocity_2>"

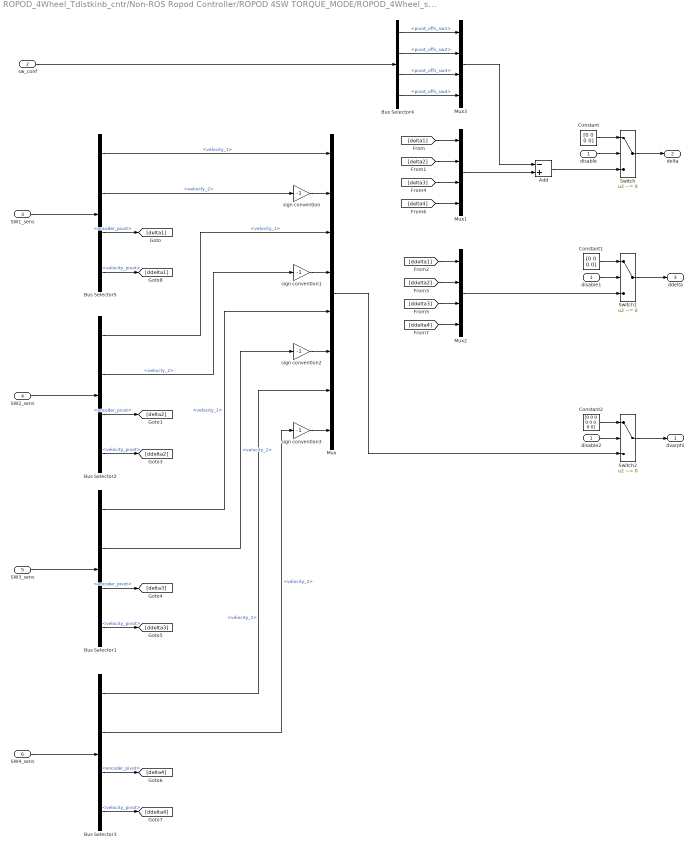
== system ROPOD_4Wheel_Tdistkinb_cntr/Non-ROS Ropod Controller/ROPOD 4SW TORQUE_MODE/ROPOD_4Wheel_sens_old ==
  disable : Inport
  sw_conf : Inport  Port=2
  SW1_sens : Inport  Port=3
  SW2_sens : Inport  Port=4
  SW3_sens : Inport  Port=5
  SW4_sens : Inport  Port=6
  Add : Sum  Inputs=-+
  Bus Selector{1..3,5} (4 alike) : BusSelector  OutputSignals=velocity_1,velocity_2,encoder_pivot,velocity_pivot
  Bus Selector4 : BusSelector  OutputSignals=pivot_offs_sw1,pivot_offs_sw2,pivot_offs_sw3,pivot_offs_sw4
  Constant : Constant  Value=[0 0 0 0]
  Constant1 : Constant  Value=[0 0 0 0]
  Constant2 : Constant  Value=[0 0 0 0 0 0 0 0]
  Mux : Mux  Inputs=8
  Mux1 : Mux
  Mux2 : Mux
  Mux3 : Mux
  Switch : Switch  Criteria=u2 ~= 0
  Switch1 : Switch  Criteria=u2 ~= 0
  Switch2 : Switch  Criteria=u2 ~= 0
  disable1 : InportShadow
  disable2 : InportShadow
  sign convention{,1..3} (4 alike) : Gain  Gain=-1
  dvarphi : Outport
  delta : Outport  Port=2
  ddelta : Outport  Port=3
  wires:
  SW1_sens/1 -> Bus Selector5/1
  SW2_sens/1 -> Bus Selector2/1
  Bus Selector5/1 -> Mux/1  "<velocity_1>"
  Bus Selector5/2 -> sign convention/1  "<velocity_2>"
  Bus Selector2/1 -> Mux/3  "<velocity_1>"
  Bus Selector2/2 -> sign convention1/1  "<velocity_2>"
  Bus Selector2/3 -> [delta2]  "<encoder_pivot>"
  [delta1] -> Mux1/1
  [delta2] -> Mux1/2
  Bus Selector2/4 -> [ddelta2]  "<velocity_pivot>"
  [ddelta2] -> Mux2/2
  [ddelta1] -> Mux2/1
  Bus Selector1/4 -> [ddelta3]  "<velocity_pivot>"
  Bus Selector1/3 -> [delta3]  "<encoder_pivot>"
  Bus Selector1/2 -> sign convention2/1  "<velocity_2>"
  Bus Selector1/1 -> Mux/5  "<velocity_1>"
  SW3_sens/1 -> Bus Selector1/1
  [delta3] -> Mux1/3
  [ddelta3] -> Mux2/3
  SW4_sens/1 -> Bus Selector3/1
  Bus Selector3/1 -> Mux/7  "<velocity_1>"
  Bus Selector3/2 -> sign convention3/1  "<velocity_2>"
  Bus Selector3/3 -> [delta4]  "<encoder_pivot>"
  Bus Selector3/4 -> [ddelta4]  "<velocity_pivot>"
  [delta4] -> Mux1/4
  [ddelta4] -> Mux2/4
  Mux1/1 -> Add/2
  Mux3/1 -> Add/1
  sw_conf/1 -> Bus Selector4/1
  Bus Selector4/1 -> Mux3/1  "<pivot_offs_sw1>"
  Bus Selector4/2 -> Mux3/2  "<pivot_offs_sw2>"
  Bus Selector4/3 -> Mux3/3  "<pivot_offs_sw3>"
  Bus Selector4/4 -> Mux3/4  "<pivot_offs_sw4>"
  Bus Selector5/3 -> [delta1]  "<encoder_pivot>"
  Bus Selector5/4 -> [ddelta1]  "<velocity_pivot>"
  sign convention/1 -> Mux/2
  sign convention1/1 -> Mux/4
  sign convention2/1 -> Mux/6
  sign convention3/1 -> Mux/8
  Add/1 -> Switch/3
  Switch/1 -> delta/1
  disable/1 -> Switch/2
  Constant/1 -> Switch/1
  Switch1/1 -> ddelta/1
  Mux2/1 -> Switch1/3
  Constant1/1 -> Switch1/1
  disable1/1 -> Switch1/2
  disable2/1 -> Switch2/2
  Constant2/1 -> Switch2/1
  Mux/1 -> Switch2/3
  Switch2/1 -> dvarphi/1

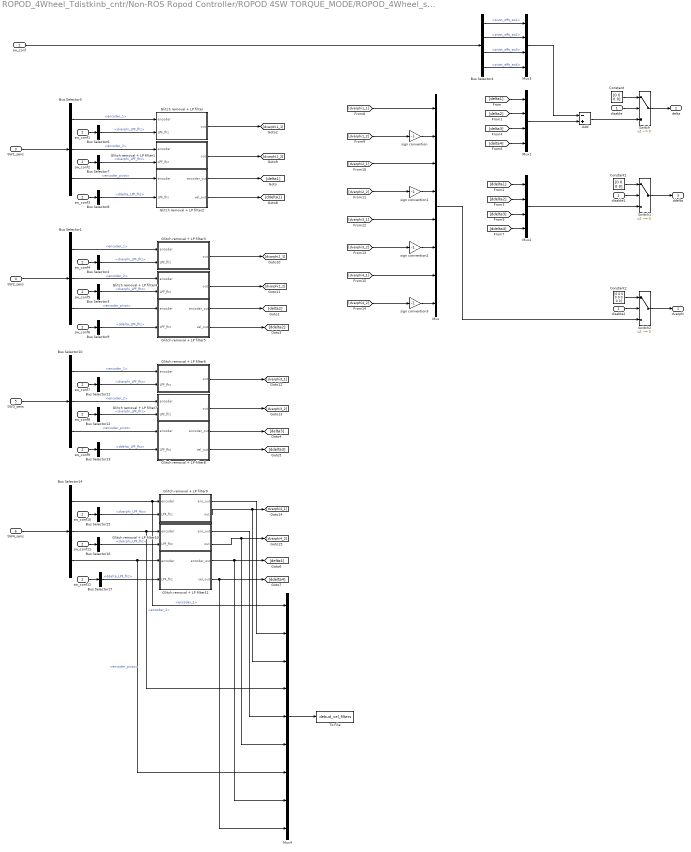
== system ROPOD_4Wheel_Tdistkinb_cntr/Non-ROS Ropod Controller/ROPOD 4SW TORQUE_MODE/ROPOD_4Wheel_sens_own_filters ==
  disable : Inport
  sw_conf : Inport  Port=2
  SW1_sens : Inport  Port=3
  SW2_sens : Inport  Port=4
  SW3_sens : Inport  Port=5
  SW4_sens : Inport  Port=6
  Add : Sum  Inputs=-+
  Bus Selector{1,5,10,14} (4 alike) : BusSelector  OutputSignals=encoder_1,encoder_2,encoder_pivot
  Bus Selector{2..3,6..7,11..12,15..16} (8 alike) : BusSelector  OutputSignals=dvarphi_LPF_fhz
  Bus Selector{8..9,13,17} (4 alike) : BusSelector  OutputSignals=ddelta_LPF_fhz
  Bus Selector4 : BusSelector  OutputSignals=pivot_offs_sw1,pivot_offs_sw2,pivot_offs_sw3,pivot_offs_sw4
  Constant : Constant  Value=[0 0 0 0]
  Constant1 : Constant  Value=[0 0 0 0]
  Constant2 : Constant  Value=[0 0 0 0 0 0 0 0]
  Glitch removal + LP filter : Subsystem
  Glitch removal + LP filter1 : Subsystem
  Glitch removal + LP filter10 : Subsystem
  Glitch removal + LP filter11 : Subsystem
  Glitch removal + LP filter2 : Subsystem
  Glitch removal + LP filter3 : Subsystem
  Glitch removal + LP filter4 : Subsystem
  Glitch removal + LP filter5 : Subsystem
  Glitch removal + LP filter6 : Subsystem
  Glitch removal + LP filter7 : Subsystem
  Glitch removal + LP filter8 : Subsystem
  Glitch removal + LP filter9 : Subsystem
  Mux : Mux  Inputs=8
  Mux1 : Mux
  Mux2 : Mux
  Mux3 : Mux
  Mux4 : Mux  Inputs=9
  Switch : Switch  Criteria=u2 ~= 0
  Switch1 : Switch  Criteria=u2 ~= 0
  Switch2 : Switch  Criteria=u2 ~= 0
  To File : ToFile  Filename=debud_vel_filters  MatrixName=debud_vel_filters
  disable1 : InportShadow
  disable2 : InportShadow
  sign convention{,1..3} (4 alike) : Gain  Gain=-1
  sw_conf{1..12} (12 alike) : InportShadow  Port=2
  dvarphi : Outport
  delta : Outport  Port=2
  ddelta : Outport  Port=3
  wires:
  SW1_sens/1 -> Bus Selector5/1
  SW2_sens/1 -> Bus Selector1/1
  [delta1] -> Mux1/1
  [delta2] -> Mux1/2
  [ddelta2] -> Mux2/2
  [ddelta1] -> Mux2/1
  SW3_sens/1 -> Bus Selector10/1
  [delta3] -> Mux1/3
  [ddelta3] -> Mux2/3
  SW4_sens/1 -> Bus Selector14/1
  [delta4] -> Mux1/4
  [ddelta4] -> Mux2/4
  Mux1/1 -> Add/2
  Mux3/1 -> Add/1
  Bus Selector4/1 -> Mux3/1  "<pivot_offs_sw1>"
  Bus Selector4/2 -> Mux3/2  "<pivot_offs_sw2>"
  Bus Selector4/3 -> Mux3/3  "<pivot_offs_sw3>"
  Bus Selector4/4 -> Mux3/4  "<pivot_offs_sw4>"
  Bus Selector5/3 -> Glitch removal + LP filter2/1(encoder)  "<encoder_pivot>"
  sign convention/1 -> Mux/2
  sign convention1/1 -> Mux/4
  sign convention2/1 -> Mux/6
  sign convention3/1 -> Mux/8
  Add/1 -> Switch/3
  Switch/1 -> delta/1
  disable/1 -> Switch/2
  Constant/1 -> Switch/1
  Switch1/1 -> ddelta/1
  Mux2/1 -> Switch1/3
  Constant1/1 -> Switch1/1
  disable1/1 -> Switch1/2
  disable2/1 -> Switch2/2
  Constant2/1 -> Switch2/1
  Mux/1 -> Switch2/3
  Switch2/1 -> dvarphi/1
  sw_conf/1 -> Bus Selector4/1
  sw_conf1/1 -> Bus Selector6/1
  sw_conf2/1 -> Bus Selector7/1
  sw_conf3/1 -> Bus Selector8/1
  sw_conf6/1 -> Bus Selector9/1
  sw_conf4/1 -> Bus Selector2/1
  sw_conf5/1 -> Bus Selector3/1
  sw_conf9/1 -> Bus Selector13/1
  sw_conf7/1 -> Bus Selector11/1
  sw_conf8/1 -> Bus Selector12/1
  sw_conf12/1 -> Bus Selector17/1
  sw_conf10/1 -> Bus Selector15/1
  sw_conf11/1 -> Bus Selector16/1
  [dvarphi1_1] -> Mux/1
  [dvarphi1_2] -> sign convention/1
  [dvarphi2_1] -> Mux/3
  [dvarphi2_2] -> sign convention1/1
  [dvarphi3_1] -> Mux/5
  [dvarphi3_2] -> sign convention2/1
  [dvarphi4_1] -> Mux/7
  [dvarphi4_2] -> sign convention3/1
  Mux4/1 -> To File/1
  Bus Selector5/1 -> Glitch removal + LP filter/1(encoder)  "<encoder_1>"
  Bus Selector6/1 -> Glitch removal + LP filter/2(LPF_fhz)  "<dvarphi_LPF_fhz>"
  Glitch removal + LP filter/1(out) -> [dvarphi1_1]
  Bus Selector7/1 -> Glitch removal + LP filter1/2(LPF_fhz)  "<dvarphi_LPF_fhz>"
  Bus Selector5/2 -> Glitch removal + LP filter1/1(encoder)  "<encoder_2>"
  Bus Selector8/1 -> Glitch removal + LP filter2/2(LPF_fhz)  "<ddelta_LPF_fhz>"
  Glitch removal + LP filter1/1(out) -> [dvarphi1_2]
  Glitch removal + LP filter2/1(encoder_out) -> [delta1]
  Glitch removal + LP filter2/2(vel_out) -> [ddelta1]
  Bus Selector2/1 -> Glitch removal + LP filter3/2(LPF_fhz)  "<dvarphi_LPF_fhz>"
  Bus Selector9/1 -> Glitch removal + LP filter5/2(LPF_fhz)  "<ddelta_LPF_fhz>"
  Bus Selector3/1 -> Glitch removal + LP filter4/2(LPF_fhz)  "<dvarphi_LPF_fhz>"
  Glitch removal + LP filter5/2(vel_out) -> [ddelta2]
  Glitch removal + LP filter3/1(out) -> [dvarphi2_1]
  Glitch removal + LP filter5/1(encoder_out) -> [delta2]
  Glitch removal + LP filter4/1(out) -> [dvarphi2_2]
  Bus Selector1/1 -> Glitch removal + LP filter3/1(encoder)  "<encoder_1>"
  Bus Selector1/2 -> Glitch removal + LP filter4/1(encoder)  "<encoder_2>"
  Bus Selector1/3 -> Glitch removal + LP filter5/1(encoder)  "<encoder_pivot>"
  Bus Selector13/1 -> Glitch removal + LP filter8/2(LPF_fhz)  "<ddelta_LPF_fhz>"
  Bus Selector10/1 -> Glitch removal + LP filter6/1(encoder)  "<encoder_1>"
  Glitch removal + LP filter7/1(out) -> [dvarphi3_2]
  Glitch removal + LP filter6/1(out) -> [dvarphi3_1]
  Bus Selector12/1 -> Glitch removal + LP filter7/2(LPF_fhz)  "<dvarphi_LPF_fhz>"
  Bus Selector10/3 -> Glitch removal + LP filter8/1(encoder)  "<encoder_pivot>"
  Glitch removal + LP filter8/1(encoder_out) -> [delta3]
  Glitch removal + LP filter8/2(vel_out) -> [ddelta3]
  Bus Selector11/1 -> Glitch removal + LP filter6/2(LPF_fhz)  "<dvarphi_LPF_fhz>"
  Bus Selector10/2 -> Glitch removal + LP filter7/1(encoder)  "<encoder_2>"
  Bus Selector17/1 -> Glitch removal + LP filter11/2(LPF_fhz)  "<ddelta_LPF_fhz>"
  Bus Selector14/1 -> Mux4/1, Glitch removal + LP filter9/1(encoder)  "<encoder_1>"
  Glitch removal + LP filter10/2(out) -> Mux4/6, [dvarphi4_2]
  Glitch removal + LP filter9/2(out) -> [dvarphi4_1], Mux4/3
  Bus Selector16/1 -> Glitch removal + LP filter10/2(LPF_fhz)  "<dvarphi_LPF_fhz>"
  Bus Selector14/3 -> Mux4/7, Glitch removal + LP filter11/1(encoder)  "<encoder_pivot>"
  Glitch removal + LP filter11/1(encoder_out) -> Mux4/8, [delta4]
  Glitch removal + LP filter11/2(vel_out) -> Mux4/9, [ddelta4]
  Bus Selector15/1 -> Glitch removal + LP filter9/2(LPF_fhz)  "<dvarphi_LPF_fhz>"
  Bus Selector14/2 -> Mux4/4, Glitch removal + LP filter10/1(encoder)  "<encoder_2>"
  Glitch removal + LP filter9/1(enc_out) -> Mux4/2
  Glitch removal + LP filter10/1(enc_out) -> Mux4/5

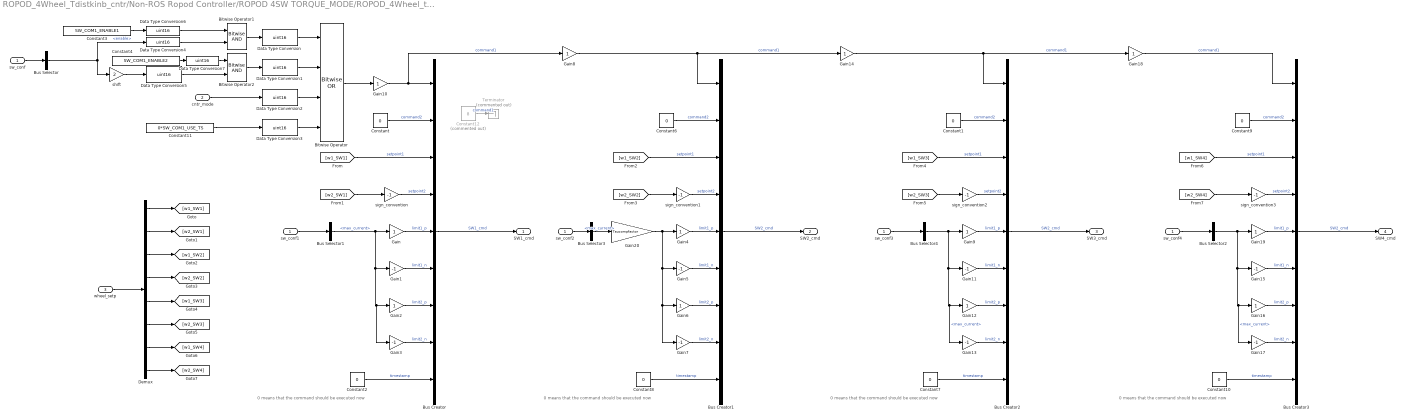
== system ROPOD_4Wheel_Tdistkinb_cntr/Non-ROS Ropod Controller/ROPOD 4SW TORQUE_MODE/ROPOD_4Wheel_torque_cmd ==
  note: 0 means that the command should be executed now
  note: 0 means that the command should be executed now
  note: 0 means that the command should be executed now
  note: 0 means that the command should be executed now
  sw_conf : Inport
  cntr_mode : Inport  Port=2
  wheel_setp : Inport  Port=3
  Bitwise Operator : simulink/Logic and Bit Operations/Bitwise Operator  logicop=OR  UseBitMask=off  NumInputPorts=4  BitMask=bin2dec('11011001')  BitMaskRealWorld=Stored Integer
  Bitwise Operator1 : simulink/Logic and Bit Operations/Bitwise Operator  logicop=AND  UseBitMask=off  NumInputPorts=2  BitMask=bin2dec('11011001')  BitMaskRealWorld=Stored Integer
  Bitwise Operator2 : simulink/Logic and Bit Operations/Bitwise Operator  logicop=AND  UseBitMask=off  NumInputPorts=2  BitMask=bin2dec('11011001')  BitMaskRealWorld=Stored Integer
  Bus Creator{,1..3} (4 alike) : BusCreator  Inputs=9
  Bus Selector : BusSelector  OutputSignals=enable
  Bus Selector{1..4} (4 alike) : BusSelector  OutputSignals=max_current
  Constant{,1..2,6..10} (8 alike) : Constant  Value=0
  Constant11 : Constant  Value=0*SW_COM1_USE_TS
  Constant12 : Constant  Commented=on  Value=8
  Constant3 : Constant  Value=SW_COM1_ENABLE1
  Constant4 : Constant  Value=SW_COM1_ENABLE2
  Data Type Conversion{,1..7} (8 alike) : DataTypeConversion  OutDataTypeStr=uint16
  Demux : Demux  Outputs=8
  Gain{,2,4,6,9,12,16,19} (8 alike) : Gain
  Gain{1,3,5,7,11,13,15,17} (8 alike) : Gain  Gain=-1
  Gain{8,10,14,18} (4 alike) : Gain  OutDataTypeStr=double
  Gain20 : Gain  Gain=Taucompfactor
  Terminator : Terminator  Commented=on
  shift : Gain  Gain=2
  sign_convention{,1..3} (4 alike) : Gain  Gain=-1
  sw_conf{1..4} (4 alike) : InportShadow
  SW1_cmd : Outport
  SW2_cmd : Outport  Port=2
  SW3_cmd : Outport  Port=3
  SW4_cmd : Outport  Port=4
  wires:
  Bus Creator/1 -> SW1_cmd/1  "SW1_cmd"
  Constant2/1 -> Bus Creator/9  "timestamp"
  Constant/1 -> Bus Creator/2  "command2"
  [w1_SW1] -> Bus Creator/3  "setpoint1"
  Bus Selector1/1 -> Gain3/1, Gain2/1, Gain1/1, Gain/1  "<max_current>"
  [w2_SW1] -> sign_convention/1
  [w2_SW2] -> sign_convention1/1
  [w1_SW2] -> Bus Creator1/3  "setpoint1"
  Constant6/1 -> Bus Creator1/2  "command2"
  Constant8/1 -> Bus Creator1/9  "timestamp"
  Bus Creator1/1 -> SW2_cmd/1  "SW2_cmd"
  Demux/4 -> [w2_SW2]
  Demux/1 -> [w1_SW1]
  Demux/2 -> [w2_SW1]
  Demux/3 -> [w1_SW2]
  wheel_setp/1 -> Demux/1
  Gain/1 -> Bus Creator/5  "limit1_p"
  Gain1/1 -> Bus Creator/6  "limit1_n"
  Gain2/1 -> Bus Creator/7  "limit2_p"
  Gain3/1 -> Bus Creator/8  "limit2_n"
  Gain6/1 -> Bus Creator1/7  "limit2_p"
  Gain4/1 -> Bus Creator1/5  "limit1_p"
  Gain5/1 -> Bus Creator1/6  "limit1_n"
  Gain7/1 -> Bus Creator1/8  "limit2_n"
  Bus Selector3/1 -> Gain20/1  "<max_current>"
  Gain8/1 -> Gain14/1, Bus Creator1/1  "command1"
  Bitwise Operator/1 -> Gain10/1
  Bitwise Operator1/1 -> Data Type Conversion/1
  Data Type Conversion2/1 -> Bitwise Operator/3
  Data Type Conversion1/1 -> Bitwise Operator/2
  Data Type Conversion3/1 -> Bitwise Operator/4
  Bitwise Operator2/1 -> Data Type Conversion1/1
  Data Type Conversion/1 -> Bitwise Operator/1
  Constant11/1 -> Data Type Conversion3/1
  sw_conf/1 -> Bus Selector/1
  Bus Selector/1 -> Data Type Conversion4/1, shift/1  "<enable>"
  sw_conf1/1 -> Bus Selector1/1
  Gain10/1 -> Bus Creator/1, Gain8/1  "command1"
  sw_conf2/1 -> Bus Selector3/1
  Gain12/1 -> Bus Creator2/7  "limit2_p"
  [w2_SW3] -> sign_convention2/1
  Bus Creator2/1 -> SW3_cmd/1  "SW2_cmd"
  Gain13/1 -> Bus Creator2/8  "limit2_n"
  sw_conf3/1 -> Bus Selector4/1
  Gain11/1 -> Bus Creator2/6  "limit1_n"
  Constant1/1 -> Bus Creator2/2  "command2"
  [w1_SW3] -> Bus Creator2/3  "setpoint1"
  Constant7/1 -> Bus Creator2/9  "timestamp"
  Bus Selector4/1 -> Gain13/1, Gain12/1, Gain11/1, Gain9/1  "<max_current>"
  Gain9/1 -> Bus Creator2/5  "limit1_p"
  Demux/5 -> [w1_SW3]
  Demux/6 -> [w2_SW3]
  Gain19/1 -> Bus Creator3/5  "limit1_p"
  Bus Selector2/1 -> Gain19/1, Gain15/1, Gain16/1, Gain17/1  "<max_current>"
  Constant10/1 -> Bus Creator3/9  "timestamp"
  [w1_SW4] -> Bus Creator3/3  "setpoint1"
  Constant9/1 -> Bus Creator3/2  "command2"
  Gain15/1 -> Bus Creator3/6  "limit1_n"
  sw_conf4/1 -> Bus Selector2/1
  Gain17/1 -> Bus Creator3/8  "limit2_n"
  Bus Creator3/1 -> SW4_cmd/1  "SW2_cmd"
  [w2_SW4] -> sign_convention3/1
  Gain16/1 -> Bus Creator3/7  "limit2_p"
  Gain18/1 -> Bus Creator3/1  "command1"
  Gain14/1 -> Gain18/1, Bus Creator2/1  "command1"
  Demux/7 -> [w1_SW4]
  Demux/8 -> [w2_SW4]
  shift/1 -> Data Type Conversion5/1
  Data Type Conversion4/1 -> Bitwise Operator1/2
  Data Type Conversion5/1 -> Bitwise Operator2/2
  Constant3/1 -> Data Type Conversion6/1
  Data Type Conversion6/1 -> Bitwise Operator1/1
  Constant4/1 -> Data Type Conversion7/1
  Data Type Conversion7/1 -> Bitwise Operator2/1
  sign_convention/1 -> Bus Creator/4  "setpoint2"
  sign_convention1/1 -> Bus Creator1/4  "setpoint2"
  sign_convention2/1 -> Bus Creator2/4  "setpoint2"
  sign_convention3/1 -> Bus Creator3/4  "setpoint2"
  Constant12/1 -> Terminator/1  "command1"
  cntr_mode/1 -> Data Type Conversion2/1
  Gain20/1 -> Gain7/1, Gain6/1, Gain5/1, Gain4/1
